simulink model "Final_RL_Load_2022a"  (R2024a)
settings: Solver=ode23tb  StartTime=0.0  StopTime=0.02  MaxStep=1E-5  MinStep=1E-6  RelTol=1e-3
libraries: nesl_utility x17, fl_lib x16, ee_lib x6, simulink x1
settings Model: Creator=Kaliamoorthy  LastModifiedBy=admin
settings RTWCC: GPUComputeCapability=3.5

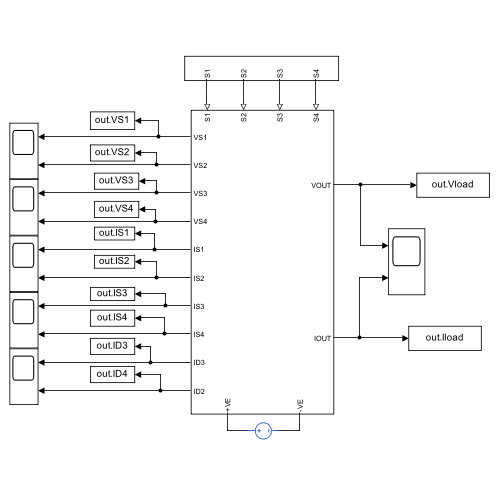
[thumbnail: Simulink's stored preview of the top-level diagram]
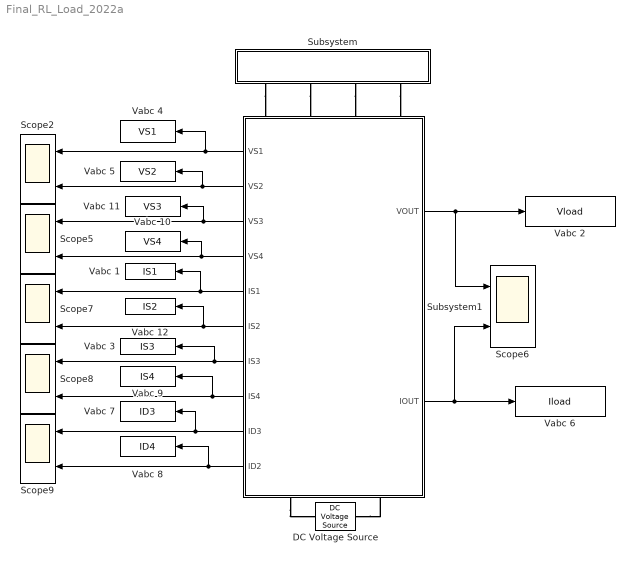
== system Final_RL_Load_2022a ==
  DC Voltage Source : fl_lib/Electrical/Electrical Sources/DC Voltage Source  v0=100 V
  Scope{2,5..9} (6 alike) : Scope  NumInputPorts=2
  Subsystem : Subsystem
  Subsystem1 : Subsystem
      settings: PortSchema="{\"entries\":[{\"content\":{\"sides\":[{\"content\":{\"connectorIds\":[\"Out3\",\"Out4\",\"Out5\",\"Out6\",\"Out7\",\"Out8\",\"Out9\",\"Out10\",\"Out11\",\"Out12\"]},\"type\":\"ConnectorPlacement.EquallySpacedRectSide\",\"uuid\":\"5d4c92a2-ca5b-4360-96e8-41c3d64711ed\"},{\"content\":{\"connectorIds\":[\"Out1\",\"Out2\"],\"side\":\"RIGHT\"},\"type\":\"ConnectorPlacement.EquallySpacedRectSide\",\"uuid\":\"a457f45b-9620-4720-a303-64053e00b06b\"},{\"content\":{\"connectorIds\":[\"LConn1\",\"LConn2\",\"LConn3\",\"LConn4\"],\"side\":\"TOP\"},\"type\":\"ConnectorPlacement.EquallySpacedRectSide\",\"uuid\":\"298cbb4c-8ecf-4ea0-bed4-5b126e4f88f2\"},{\"content\":{\"connectorIds\":[\"RConn1\",\"RConn2\"],\"side\":\"BOTTOM\"},\"type\":\"ConnectorPlacement.EquallySpacedRectSide\",\"uuid\":\"7f9a027b-cc9b-4311-87e5-9c4d634c220b\"}]},\"type\":\"ConnectorPlacement.EquallySpacedConnector\",\"uuid\":\"e00c9d97-7469-4c00-8f13-230a23b74654\"}],\"packageUris\":[\"http://schema.mathworks.com/mf0/Connector/R2020b\"],\"version\":\"1.0\"}"
  Vabc 1 : ToWorkspace  VariableName=IS1  SaveFormat=Timeseries  SampleTime=-1
  Vabc 10 : ToWorkspace  VariableName=VS4  SaveFormat=Timeseries  SampleTime=-1
  Vabc 11 : ToWorkspace  VariableName=VS3  SaveFormat=Timeseries  SampleTime=-1
  Vabc 12 : ToWorkspace  VariableName=IS2  SaveFormat=Timeseries  SampleTime=-1
  Vabc 2 : ToWorkspace  VariableName=Vload  SaveFormat=Timeseries  SampleTime=-1
  Vabc 3 : ToWorkspace  VariableName=IS3  SaveFormat=Timeseries  SampleTime=-1
  Vabc 4 : ToWorkspace  VariableName=VS1  SaveFormat=Timeseries  SampleTime=-1
  Vabc 5 : ToWorkspace  VariableName=VS2  SaveFormat=Timeseries  SampleTime=-1
  Vabc 6 : ToWorkspace  VariableName=Iload  SaveFormat=Timeseries  SampleTime=-1
  Vabc 7 : ToWorkspace  VariableName=ID3  SaveFormat=Timeseries  SampleTime=-1
  Vabc 8 : ToWorkspace  VariableName=ID4  SaveFormat=Timeseries  SampleTime=-1
  Vabc 9 : ToWorkspace  VariableName=IS4  SaveFormat=Timeseries  SampleTime=-1
  wires:
  Subsystem1/1(VOUT) -> Vabc 2/1, Scope6/1
  Subsystem1/2(IOUT) -> Scope6/2, Vabc 6/1
  Subsystem1/3(VS1) -> Vabc 4/1, Scope2/1
  Subsystem1/4(VS2) -> Vabc 5/1, Scope2/2
  Subsystem1/5(VS3) -> Vabc 11/1, Scope5/1
  Subsystem1/6(VS4) -> Vabc 10/1, Scope5/2
  Subsystem1/7(IS1) -> Vabc 1/1, Scope7/1
  Subsystem1/8(IS2) -> Vabc 12/1, Scope7/2
  Subsystem1/10(IS4) -> Vabc 9/1, Scope8/2
  Subsystem1/9(IS3) -> Vabc 3/1, Scope8/1
  Subsystem1/11(ID3) -> Vabc 7/1, Scope9/1
  Subsystem1/12(ID2) -> Vabc 8/1, Scope9/2
  connections:
  Subsystem1/RConn1 -- DC Voltage Source/LConn1
  DC Voltage Source/RConn1 -- Subsystem1/RConn2
  Subsystem/RConn1 -- Subsystem1/LConn1
  Subsystem/RConn2 -- Subsystem1/LConn2
  Subsystem/RConn3 -- Subsystem1/LConn3
  Subsystem/RConn4 -- Subsystem1/LConn4

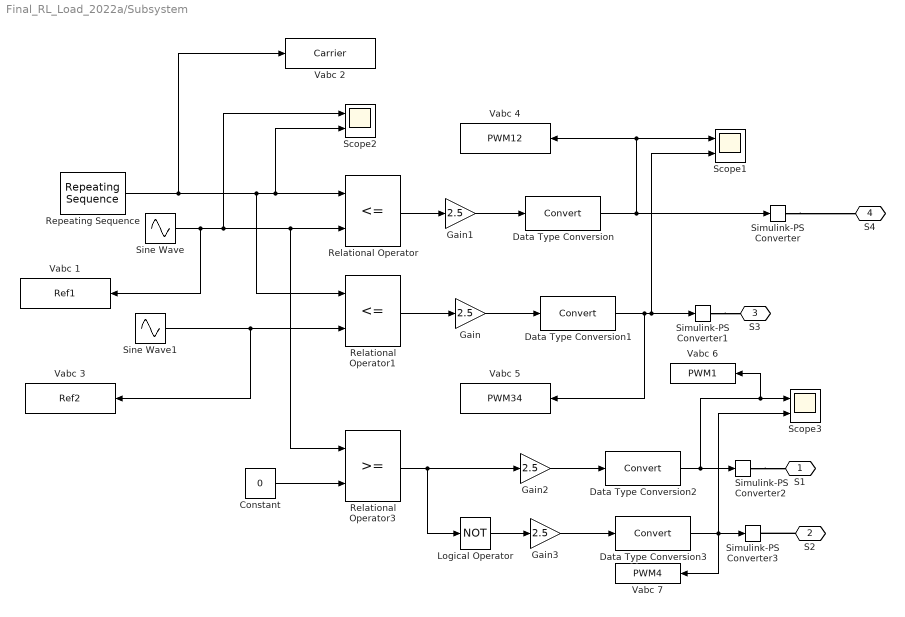
== system Final_RL_Load_2022a/Subsystem ==
  Constant : Constant  Value=0
  Data Type Conversion{,1..3} (4 alike) : DataTypeConversion  SaturateOnIntegerOverflow=off  RndMeth=Floor
  Gain{,1..3} (4 alike) : Gain  Gain=2.5
  Logical Operator : Logic  Operator=NOT  AllPortsSameDT=off  OutDataTypeStr=boolean
  Relational Operator : RelationalOperator  Operator=<=  OutDataTypeStr=boolean  RndMeth=Simplest  InputSameDT=off
  Relational Operator1 : RelationalOperator  Operator=<=  OutDataTypeStr=boolean  RndMeth=Simplest  InputSameDT=off
  Relational Operator3 : RelationalOperator  OutDataTypeStr=boolean  RndMeth=Simplest  InputSameDT=off
  Repeating Sequence : simulink/Sources/Repeating Sequence  rep_seq_t=[0 (1/1000)/2 1/1000]  rep_seq_y=[0 1 0]
  Scope1 : Scope  NumInputPorts=2
  Scope2 : Scope  NumInputPorts=2
  Scope3 : Scope  NumInputPorts=2
  Simulink-PS Converter{,1..3} (4 alike) : nesl_utility/Simulink-PS Converter  PhysicalDomain=network_engine_domain  SubClassName=ps_input  LeftPortType=input  RightPortType=output  PseudoPeriodic=off  Frequencies=[]  NoiseDistribution=none  NoiseParameters=[]  Unit=1  AffineConversion=off  FilteringAndDerivatives=provide  SimscapeFilterOrder=1  InputFilterTimeConstant=0.001  UdotUserProvided=0
  Sine Wave : Sin  Amplitude=0.9  Frequency=2*pi*50  SampleTime=0
  Sine Wave1 : Sin  Amplitude=0.9  Frequency=2*pi*50  Phase=pi  SampleTime=0
  Vabc 1 : ToWorkspace  VariableName=Ref1  SaveFormat=Timeseries  SampleTime=-1
  Vabc 2 : ToWorkspace  VariableName=Carrier  SaveFormat=Timeseries  SampleTime=-1
  Vabc 3 : ToWorkspace  VariableName=Ref2  SaveFormat=Timeseries  SampleTime=-1
  Vabc 4 : ToWorkspace  VariableName=PWM12  SaveFormat=Timeseries  SampleTime=-1
  Vabc 5 : ToWorkspace  VariableName=PWM34  SaveFormat=Timeseries  SampleTime=-1
  Vabc 6 : ToWorkspace  VariableName=PWM1  SaveFormat=Timeseries  SampleTime=-1
  Vabc 7 : ToWorkspace  VariableName=PWM4  SaveFormat=Timeseries  SampleTime=-1
  S1 : PMIOPort  Side=Right
  S2 : PMIOPort  Port=2  Side=Right
  S3 : PMIOPort  Port=3  Side=Right
  S4 : PMIOPort  Port=4  Side=Right
  wires:
  Relational Operator/1 -> Gain1/1
  Sine Wave1/1 -> Vabc 3/1, Relational Operator1/2
  Sine Wave/1 -> Vabc 1/1, Scope2/1, Relational Operator3/1, Relational Operator/2
  Repeating Sequence/1 -> Vabc 2/1, Relational Operator1/1, Scope2/2, Relational Operator/1
  Relational Operator1/1 -> Gain/1
  Data Type Conversion/1 -> Scope1/1, Vabc 4/1, Simulink-PS Converter/1
  Data Type Conversion1/1 -> Vabc 5/1, Scope1/2, Simulink-PS Converter1/1
  Gain1/1 -> Data Type Conversion/1
  Gain/1 -> Data Type Conversion1/1
  Constant/1 -> Relational Operator3/2
  Gain2/1 -> Data Type Conversion2/1
  Relational Operator3/1 -> Gain2/1, Logical Operator/1
  Data Type Conversion2/1 -> Vabc 6/1, Scope3/1, Simulink-PS Converter2/1
  Gain3/1 -> Data Type Conversion3/1
  Data Type Conversion3/1 -> Vabc 7/1, Scope3/2, Simulink-PS Converter3/1
  Logical Operator/1 -> Gain3/1
  connections:
  Simulink-PS Converter1/RConn1 -- S3/RConn1
  Simulink-PS Converter/RConn1 -- S4/RConn1
  Simulink-PS Converter2/RConn1 -- S1/RConn1
  S2/RConn1 -- Simulink-PS Converter3/RConn1

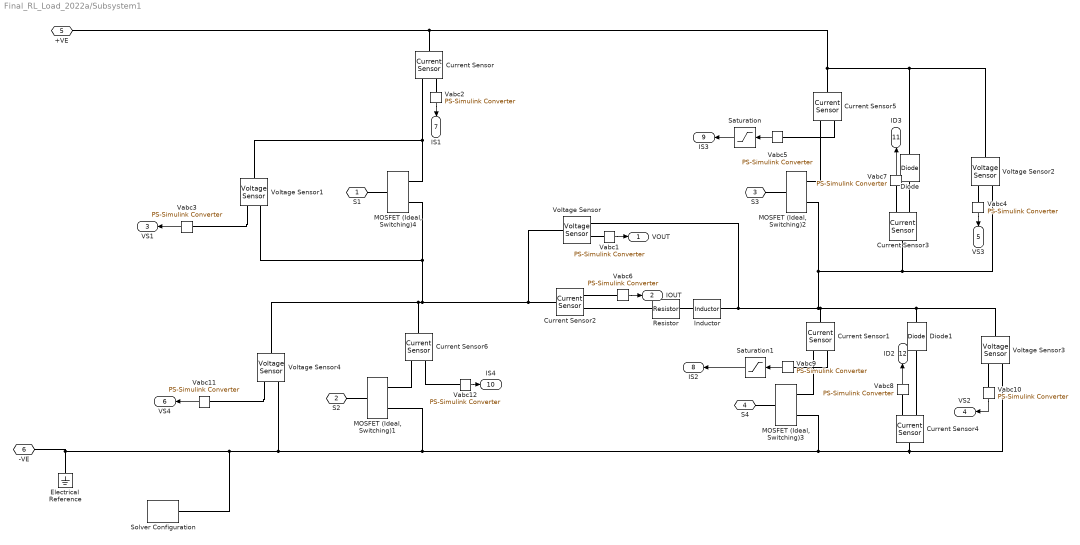
== system Final_RL_Load_2022a/Subsystem1 ==
  Current Sensor{,1..6} (7 alike) : fl_lib/Electrical/Electrical Sensors/Current Sensor
  Diode : fl_lib/Electrical/Electrical Elements/Diode  Vf=0.6 V  Ron=0.3 Ohm  Goff=1e-8 1/Ohm  i_specify=off  i_priority=None  i=0 A  i_nominal_specify=off  i_nominal_value=1  i_nominal_unit=A  v_specify=off  v_priority=None  v=0 V  v_nominal_specify=off  v_nominal_value=1  v_nominal_unit=V
  Diode1 : fl_lib/Electrical/Electrical Elements/Diode  Vf=0.6 V  Ron=0.3 Ohm  Goff=1e-8 1/Ohm  i_specify=off  i_priority=None  i=0 A  i_nominal_specify=off  i_nominal_value=1  i_nominal_unit=A  v_specify=off  v_priority=None  v=0 V  v_nominal_specify=off  v_nominal_value=1  v_nominal_unit=V
  Electrical Reference : fl_lib/Electrical/Electrical Elements/Electrical Reference
  Inductor : ee_lib/Passive/Inductor  l=50 mH  enable_L_tol=ee.enum.toleranceApplication.none  L_tol=20  tol_distribution=ee.enum.toleranceDistribution.uniform  nSigma=4  r=0 Ohm  g=1e-9 1/Ohm  enable_operating_limits=ee.enum.enable.no  operating_limit_action=ee.enum.passive.reportOpLim.warn  max_working_current=1 A  power_rating=1 W  enable_faults=ee.enum.enable.no  fault_action=simscape.enum.assert.action.none  lambdaPercent=50  k_faulted=0.9999  turnsShort=ee.enum.passive.inductor.turnsShortOption.no  openCct=ee.enum.enable.no  groundShort=ee.enum.passive.inductor.groundShortOption.no  groundShortG=0 1/Ohm  tau_fault=1e-3 s  fault_trigger=ee.enum.faults.faultTrigger.temporal  t_fault=1 s  max_permissible_voltage=100 V  n_fail_on_voltage=1  max_permissible_current=1 A  t_fail_on_current=1 s  i_L_specify=off  i_L_priority=High  i_L=0 A  i_L_nominal_specify=off  i_L_nominal_value=1  i_L_nominal_unit=A  faulted_specify=off  faulted_priority=None  faulted=0
  MOSFET (Ideal, Switching){1..4} (4 alike) : ee_lib/Semiconductors & Converters/MOSFET (Ideal, Switching)  port_option=ee.enum.controlport.ps  Rds=0.01 Ohm  Goff=1e-6 1/Ohm  Vth=2 V  diode_param=ee.enum.converters.protectiondiode.none  diode_Vf=0.8 V  diode_Ron=0.001 Ohm  diode_Goff=1e-5 1/Ohm  diode_C=50e-9 F  diode_iRM=-235 A  diode_iF=300 A  diode_idot=-50 A/us  diode_trr_param=ee.enum.converters.diodeReverseParam.trr_factor  diode_trr_factor=3  diode_trr=15 us  diode_Qrr=1500 s*uA  ids_specify=off  ids_priority=None  ids=0 A  ids_nominal_specify=off  ids_nominal_value=1  ids_nominal_unit=A  vds_specify=off  vds_priority=None  vds=0 V  vds_nominal_specify=off  vds_nominal_value=1  vds_nominal_unit=V  vgs_specify=off  vgs_priority=None  vgs=0 V  vgs_nominal_specify=off  vgs_nominal_value=1  vgs_nominal_unit=V  thermal_loss_option=ee.enum.converters.thermalLossOption.constantvalues  Von_data=[0, 1.8, 3.2, 6, 10, 16; 0, 2, 5.5, 9.5, 15, 25] V  Tj=[298.15, 448.15] K  Iout_data=[0, 20, 40, 60, 80, 100] A  Eon_data=[0, 55.04, 124.57, 235.53, 362.12; 0, 71.25, 161.25, 304.88, 468.75] * 1e-6 J  Eoff_data=[0, 18, 30, 56.1, 76.5; 0, 22.5, 37.5, 70.13, 95.63] * 1e-6 J  Eon_data_3D=[zeros(2, 5, 3)] J  Eoff_data_3D=[zeros(2, 5, 3)] J  Tj_loss=[298.15, 448.15] K  Iout_data_loss=[0, 10, 20, 30, 40] A  tabulateWithVds=false  Vds_loss=[0, 150, 300] V  Eon_scalar=22.86e-3 J  Eoff_scalar=17.14e-3 J  Voff=300 V  Iout_scalar=600 A  useCurrentFromPreviousCycle=false  useVoltageFromPreviousCycle=false  diodeModelType=ee.enum.converters.diodeModelType.pwl  diodeTableType=ee.enum.diode.tableType.IfMat  diode_ReverseIVType=ee.enum.diode.diodeReverseIV.constant  diode_IfMat=[.07, .12, .19, 1.75, 4.24, 7.32, 11.2; .16, .3, .72, 2.14, 4.02, 6.35, 9.12] A  diode_VfMat=[.9, 1.15, 1.25, 1.5, 1.75, 2.17, 2.6, 2.85; .58, .68, .75, 1.1, 1.38, 1.77, 2.27, 2.7] V  diode_TjVec=[25, 125] degC  diode_VfVec=[.5, .7, .9, 1.3, 1.7, 2.1, 2.5] V  diode_IfVec=[.1, .2, .5, 1, 2, 4, 7, 10] A  diode_IrMat=[1e-06, 2e-06, 5e-06, 1e-05, 2.5e-05, 5e-05, .0001; 2e-06, 5e-06, 1e-05, 4e-05, 8e-05, .0002, .0005] A  diode_VrMat=[10, 100, 200, 250, 300, 325, 350; 10, 70, 160, 220, 270, 300, 320] V  diode_VrVec=[10, 20, 40, 50, 70, 80, 100] V  diode_IrVec=[1e-06, 2e-06, 5e-06, 1e-05, 2e-05, 5e-05, .0001] A  diode_Vr=-600 V  diode_Ls=150 nH  diode_Erec=0.03 J  diode_rec_loss_model=ee.enum.diode.reverseRecoveryModel.fixed  diode_ErecVal=0 J  diode_scaleWithIandV=true  diode_ErecMat=zeros(2, 3) J  diode_TjrecVec=[298.15, 398.15] K  diode_IfrecVec=[.1, 1, 10] A  diode_IrecVal=10 A  diode_VrecVal=10 V  diode_tFilter=1 / 1000 / 100 s  thermal_network_parameterization=ee.enum.thermalNetworkTopology.external  Rth=[.03, .2] K/W  Rth_Cauer=[.03, .1, .2] K/W  Rth_Foster=[.03, .2] K/W  thermal_mass_parameterization=ee.enum.thermalNetwork.timeconstant  thermal_mass=[3, 25] J/K  thermal_mass_Cauer=[3, 10, 25] J/K  thermal_mass_Foster=[33, 50] J/K  thermal_time_constant=[.1, 5] s  thermal_time_constant_Cauer=[.1, 1, 5] s  thermal_time_constant_Foster=[1, 10] s  thermal_mass_initial_temperatures=[25, 25] degC  thermal_mass_initial_temperatures_Cauer=[25, 25, 25] degC  junction_thermal_mass=0.1 J/K  Tvec_initial_Foster=[25, 25, 25, 25] degC  no_thermal_network=0  junction_temperature_specify=off  junction_temperature_priority=None  junction_temperature=25 degC  junction_temperature_nominal_specify=off  junction_temperature_nominal_value=1  junction_temperature_nominal_unit=degC  Qj_specify=off  Qj_priority=None  Qj=0 W  Qj_nominal_specify=off  Qj_nominal_value=1  Qj_nominal_unit=W  accumulatedSwitchingLosses_specify=off  accumulatedSwitchingLosses_priority=None  accumulatedSwitchingLosses=0 J
  Resistor : ee_lib/Passive/Resistor  R=125 Ohm  enable_R_tol=0  R_tol=5  tol_distribution=1  nSigma=4  enable_operating_limits=0  operating_limit_action=2  power_rating=1 W  max_working_voltage=100 V  enable_faults=ee.enum.enable.no  fault_action=simscape.enum.assert.action.none  R_faulted=inf Ohm  fault_trigger=ee.enum.faults.faultTrigger.temporal  t_fault=1 s  max_permissible_current=1 A  t_fail_on_current=1 s  noise_mode=0  Tdevice=25 degC  sample_time=1e-3 s  repeatability=1  user_seed=0  auto_seed=3499211588  faulted_specify=off  faulted_priority=None  faulted=0  power_derating_T1=70 degC  power_derating_T2=155 degC  operating_temperature_range_vec=[-50, 150] degC  alpha=3.93e-3 1/K  Tmeas=25 degC  thermal_mass=100 J/K  temperature_specify=off  temperature_priority=High  temperature=298.15 K  temperature_nominal_specify=off  temperature_nominal_value=1  temperature_nominal_unit=K
  Saturation : Saturate  UpperLimit=1  LowerLimit=-1
  Saturation1 : Saturate  UpperLimit=1  LowerLimit=-1
  Solver Configuration : nesl_utility/Solver Configuration  PhysicalDomain=network_engine_domain  SubClassName=solver  LeftPortType=input  RightPortType=generic  Tones=[]  Harmonics=[]  SimulateNoise=off  Profile=off  UseLocalSampling=off  EnableSwitchedLinearOptims=on  FrequencyDomain=off  UseCCode=off  RelTol=0.001  AbsTol=0.001  MinStep=1e-09  ToWorkspace=off  RevertToSquareIcSolve=off  NumHomotopyIterations=100  PhasorMode=off  PhasorModeNumHarmonics=1  ConsistencySolver=NEWTON_FTOL  IndexReductionMethod=DerivativeReplacement  DoDC=off  ResidualTolerance=1e-09  ConsistencyTolSource=GLOBAL  ConsistencyAbsTol=0.001  ConsistencyRelTol=0.001  ConsistencyTolFactor=0.001  UseLocalSolver=off  LocalSolverChoice=NE_BACKWARD_EULER_ADVANCER  ResolveIndetEquations=on  FunctionEvalNumThread=1  LocalSolverSampleTime=0.001  DoFixedCost=off  MaxNonlinIter=3  MaxModeIter=2  ComputeImpulses=off  ImpulseIterations=2  LinearAlgebra=auto  LinearAlgebraNumThread=0  EquationFormulation=NE_TIME_EF  DelaysMemoryBudget=1024  AutomaticFiltering=on  FilteringTimeConstant=0.001  PartitionStorageMethod=AS_NEEDED  PartitionMemoryBudget=1024  PartitionMethod=ROBUST  MultibodyUseLocalSolver=off  MultibodyLocalSolverChoice=ODE1  MultibodyLocalSolverSampleTime=0.001
  Vabc{1..12} (12 alike) : nesl_utility/PS-Simulink Converter  PhysicalDomain=network_engine_domain  SubClassName=ps_output  LeftPortType=input  RightPortType=output  PseudoPeriodic=off  Frequencies=[]  VectorFormat=inherit  Unit=inherit  AffineConversion=off
  Voltage Sensor{,1..4} (5 alike) : fl_lib/Electrical/Electrical Sensors/Voltage Sensor
  S1 : PMIOPort  Side=Left
  S2 : PMIOPort  Port=2  Side=Left
  S3 : PMIOPort  Port=3  Side=Left
  S4 : PMIOPort  Port=4  Side=Left
  +VE : PMIOPort  Port=5  Side=Right
  -VE : PMIOPort  Port=6  Side=Right
  VOUT : Outport
  IOUT : Outport  Port=2
  VS1 : Outport  Port=3
  VS2 : Outport  Port=4
  VS3 : Outport  Port=5
  VS4 : Outport  Port=6
  IS1 : Outport  Port=7
  IS2 : Outport  Port=8
  IS3 : Outport  Port=9
  IS4 : Outport  Port=10
  ID3 : Outport  Port=11
  ID2 : Outport  Port=12
  wires:
  Vabc2/1 -> IS1/1
  Vabc4/1 -> VS3/1
  Vabc1/1 -> VOUT/1
  Vabc6/1 -> IOUT/1
  Vabc5/1 -> Saturation/1
  Vabc3/1 -> VS1/1
  Vabc7/1 -> ID3/1
  Vabc8/1 -> ID2/1
  Saturation/1 -> IS3/1
  Vabc9/1 -> Saturation1/1
  Vabc11/1 -> VS4/1
  Vabc12/1 -> IS4/1
  Saturation1/1 -> IS2/1
  Vabc10/1 -> VS2/1
  connections:
  Voltage Sensor/LConn1 -- Current Sensor2/LConn1 -- Current Sensor6/LConn1 -- Voltage Sensor4/LConn1 -- "MOSFET (Ideal, Switching)4"/RConn2 -- Voltage Sensor1/RConn2
  -VE/RConn1 -- Electrical Reference/LConn1 -- Solver Configuration/RConn1 -- Voltage Sensor3/RConn2 -- Current Sensor4/LConn1 -- "MOSFET (Ideal, Switching)3"/RConn2 -- "MOSFET (Ideal, Switching)1"/RConn2 -- Voltage Sensor4/RConn2
  Inductor/LConn1 -- Resistor/RConn1
  Voltage Sensor2/LConn1 -- Diode/RConn1 -- Current Sensor5/LConn1 -- Current Sensor/LConn1 -- +VE/RConn1
  Vabc3/LConn1 -- Voltage Sensor1/RConn1
  Current Sensor3/LConn1 -- Voltage Sensor2/RConn2 -- "MOSFET (Ideal, Switching)2"/RConn2 -- Inductor/RConn1 -- Voltage Sensor/RConn2 -- Voltage Sensor3/LConn1 -- Diode1/RConn1 -- Current Sensor1/LConn1
  Current Sensor/RConn2 -- Voltage Sensor1/LConn1 -- "MOSFET (Ideal, Switching)4"/RConn1
  Vabc4/LConn1 -- Voltage Sensor2/RConn1
  "MOSFET (Ideal, Switching)4"/LConn1 -- S1/RConn1
  Vabc1/LConn1 -- Voltage Sensor/RConn1
  Current Sensor2/RConn2 -- Resistor/LConn1
  Vabc6/LConn1 -- Current Sensor2/RConn1
  Vabc2/LConn1 -- Current Sensor/RConn1
  "MOSFET (Ideal, Switching)2"/LConn1 -- S3/RConn1
  "MOSFET (Ideal, Switching)1"/LConn1 -- S2/RConn1
  "MOSFET (Ideal, Switching)3"/LConn1 -- S4/RConn1
  Current Sensor3/RConn2 -- Diode/LConn1
  Current Sensor4/RConn2 -- Diode1/LConn1
  Vabc7/LConn1 -- Current Sensor3/RConn1
  Vabc8/LConn1 -- Current Sensor4/RConn1
  Current Sensor5/RConn2 -- "MOSFET (Ideal, Switching)2"/RConn1
  Vabc5/LConn1 -- Current Sensor5/RConn1
  Vabc9/LConn1 -- Current Sensor1/RConn1
  Current Sensor1/RConn2 -- "MOSFET (Ideal, Switching)3"/RConn1
  Vabc10/LConn1 -- Voltage Sensor3/RConn1
  Vabc11/LConn1 -- Voltage Sensor4/RConn1
  Vabc12/LConn1 -- Current Sensor6/RConn1
  Current Sensor6/RConn2 -- "MOSFET (Ideal, Switching)1"/RConn1
